simulink model "simulink_04"  (R2023b)
settings: Solver=VariableStepAuto  StartTime=0.0  StopTime=10000  RelTol=1e-3
settings Model: Creator=HP  LastModifiedBy=HP

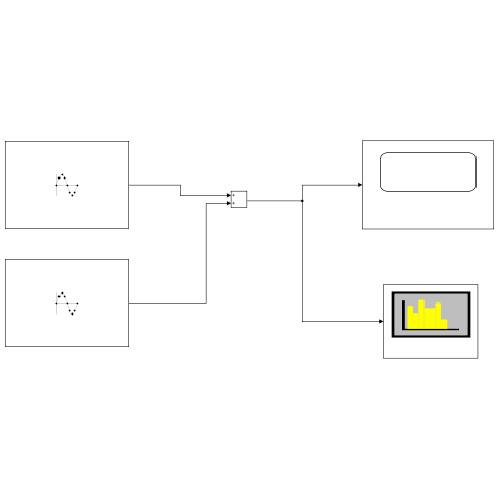
[thumbnail: Simulink's stored preview of the top-level diagram]
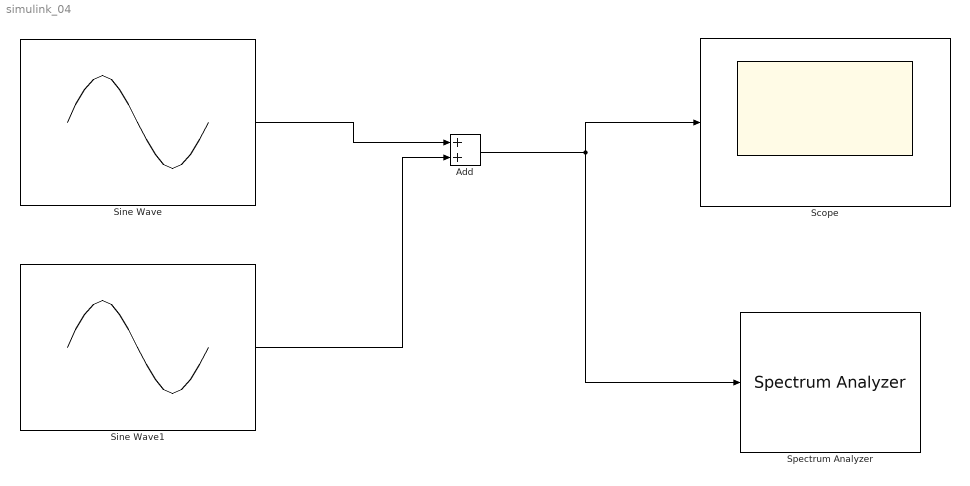
== system simulink_04 ==
  Add : Sum
  Scope : Scope
  Sine Wave : Sin  SineType=Sample based  SampleTime=1
  Sine Wave1 : Sin  SineType=Sample based  SampleTime=1  Offset=2
  Spectrum Analyzer : SpectrumAnalyzer  WindowPosition=[8.000000,22.000000,481.000000,500.000000,]  ScopeFrameLocation=window  Span=1  StartFrequency=-0.5  StopFrequency=0.5  YLimits=[-59.65627074,30.9254298]  SelectedToolstripTab=spectrumAnalyzerToolstrip.measurementsTab
  wires:
  Sine Wave/1 -> Add/1
  Add/1 -> Spectrum Analyzer/1, Scope/1
  Sine Wave1/1 -> Add/2
